simulink model "Design"  (R2024a)
settings: Solver=VariableStepAuto  StartTime=0.0  StopTime=10.0  RelTol=1e-3
libraries: RCTblocks x8
settings Model: Creator=Thoma  LastModifiedBy=Thoma

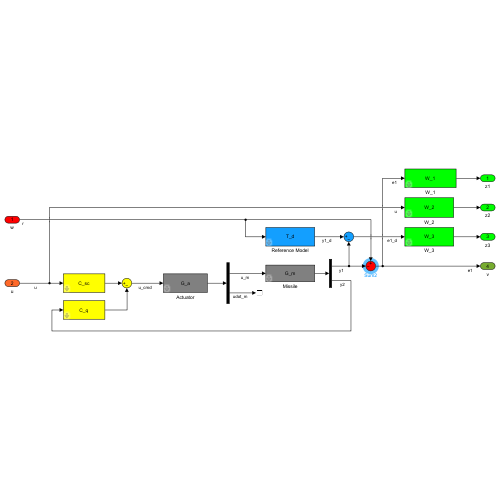
[thumbnail: Simulink's stored preview of the top-level diagram]
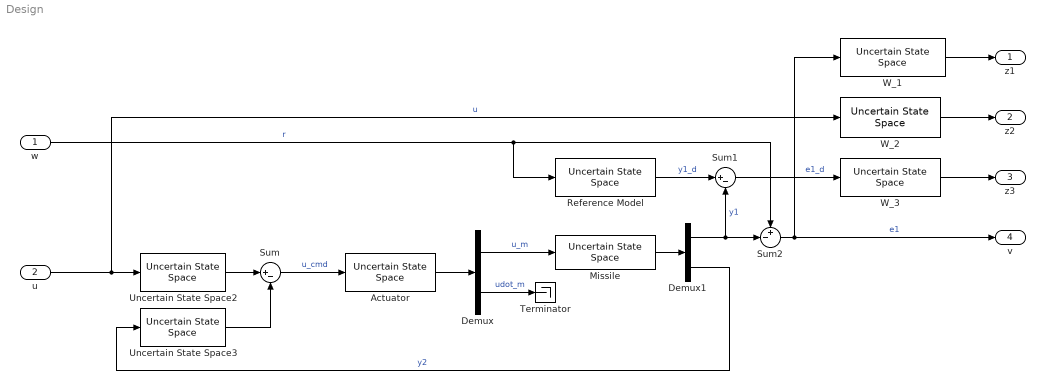
== system Design ==
  w : Inport
  u : Inport  Port=2
  Actuator : RCTblocks/Uncertain State Space  Tag=USS  USystem=G_a  UValue=[]  X0=[]  uX0=[]
  Demux : Demux  Outputs=2
  Demux1 : Demux  Outputs=2
  Missile : RCTblocks/Uncertain State Space  Tag=USS  USystem=G_m  UValue=[]  X0=[]  uX0=[]
  Reference Model : RCTblocks/Uncertain State Space  Tag=USS  USystem=T_d  UValue=[]  X0=[]  uX0=[]
  Sum : Sum  Inputs=|+-
  Sum1 : Sum  Inputs=|+-
  Sum2 : Sum  Inputs=+-|
  Terminator : Terminator
  Uncertain State Space2 : RCTblocks/Uncertain State Space  Tag=USS  USystem=C_sc  UValue=[]  X0=[]  uX0=[]
  Uncertain State Space3 : RCTblocks/Uncertain State Space  Tag=USS  USystem=C_q  UValue=[]  X0=[]  uX0=[]
  W_1 : RCTblocks/Uncertain State Space  Tag=USS  USystem=W_1  UValue=[]  X0=[]  uX0=[]
  W_2 : RCTblocks/Uncertain State Space  Tag=USS  USystem=W_2  UValue=[]  X0=[]  uX0=[]
  W_3 : RCTblocks/Uncertain State Space  Tag=USS  USystem=W_3  UValue=[]  X0=[]  uX0=[]
  z1 : Outport
  z2 : Outport  Port=2
  z3 : Outport  Port=3
  v : Outport  Port=4
  wires:
  Demux1/2 -> Uncertain State Space3/1  "y2"
  Demux/2 -> Terminator/1  "udot_m"
  Actuator/1 -> Demux/1
  Demux/1 -> Missile/1  "u_m"
  Missile/1 -> Demux1/1
  Uncertain State Space2/1 -> Sum/1
  Sum/1 -> Actuator/1  "u_cmd"
  Uncertain State Space3/1 -> Sum/2
  Demux1/1 -> Sum2/2, Sum1/2  "y1"
  u/1 -> W_2/1, Uncertain State Space2/1  "u"
  w/1 -> Sum2/1, Reference Model/1  "r"
  Reference Model/1 -> Sum1/1  "y1_d"
  Sum1/1 -> W_3/1  "e1_d"
  W_1/1 -> z1/1
  W_2/1 -> z2/1
  W_3/1 -> z3/1
  Sum2/1 -> v/1, W_1/1  "e1"
